simulink model "gm_sampleModel1655_sub"  (R2023a)
settings: Solver=VariableStepAuto  StartTime=0.0  StopTime=10.0  RelTol=1e-3
libraries: simulink x1
settings Model: Creator=user1  LastModifiedBy=user1
settings OptimizationCC: BlockReduction=off  ConditionallyExecuteInputs=off
settings DebuggingCC: InheritedTsInSrcMsg=none

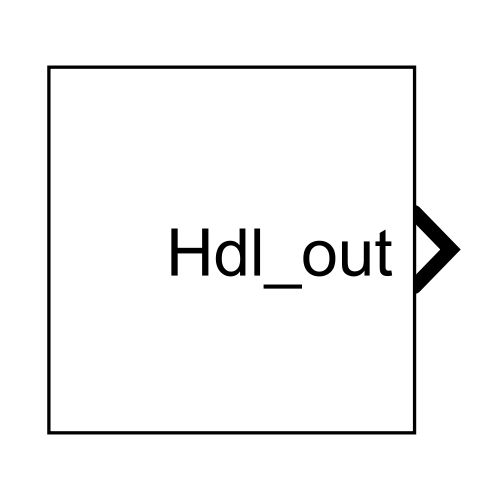
[thumbnail: Simulink's stored preview of the top-level diagram]
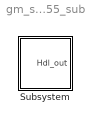
== system gm_sampleModel1655_sub ==
  Subsystem : Subsystem

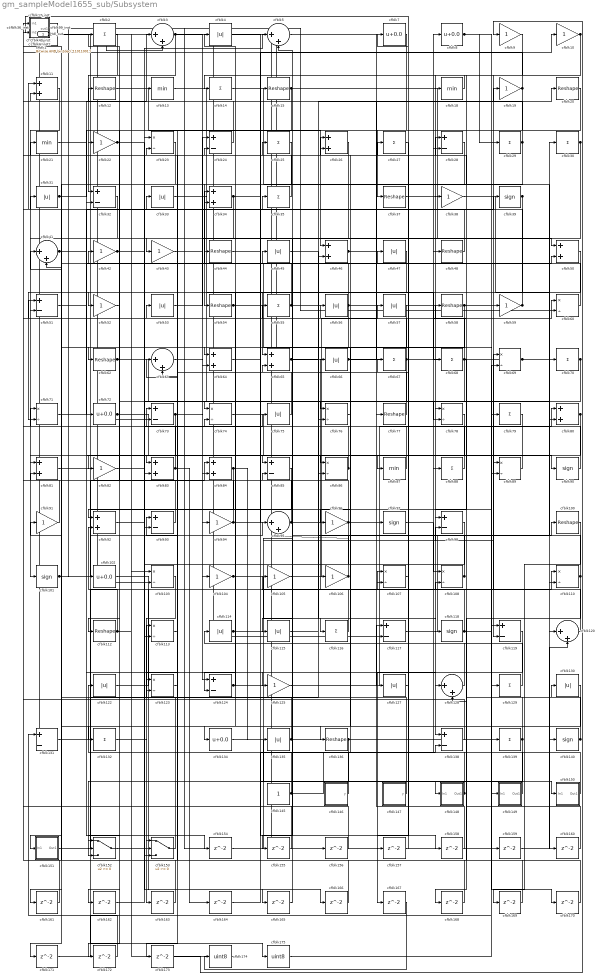
== system gm_sampleModel1655_sub/Subsystem ==
  cfblk1 : simulink/Logic and Bit Operations/Bitwise Operator  logicop=AND  UseBitMask=on  BitMask=bin2dec('11011001')  BitMaskRealWorld=Stored Integer
      settings: LibrarySourceBlock=|
      | hdlsllib/Logic and Bit
      | Operations/Bitwise
      | Operator
  cfblk{9..10,19,22,38,42..43,52,59,82,91,94,96,104..106,125} (17 alike) : Gain  OutDataTypeStr=uint8
  cfblk{12,15,20,37,44,48,54,58,62,77,100,112,136} (13 alike) : Reshape
  cfblk{39,90,97,101,118,140} (6 alike) : Signum
  cfblk{7..8,72,102,134} (5 alike) : Bias  Bias=0.0  SaturateOnIntegerOverflow=off
  cfblk{23,60,69,71,74,76,78,86,89,103,107..108,110,113,123} (15 alike) : Product  Inputs=*/  OutDataTypeStr=uint8  RndMeth=Zero  SaturateOnIntegerOverflow=on
  cfblk109_inst : Subsystem
  cfblk{11,26,34,46,50,64..65,80..81,83..84,92} (12 alike) : Sum  OutDataTypeStr=uint8
  cfblk{4,31,33,45,47,53,56..57,66,75,114..115,122,127,130,135} (16 alike) : Abs  OutDataTypeStr=uint8  SaturateOnIntegerOverflow=off
  cfblk{2,14,25,27,29..30,35,55,67..68,70,79,88,116,129,132,139} (17 alike) : Sum  Inputs=+  OutDataTypeStr=uint8
  cfblk{24,28,32,51,73,85,93,98,117,119,124,131,138} (13 alike) : Sum  Inputs=+-  OutDataTypeStr=uint8
  cfblk{3,5,41,63,95,120,128} (7 alike) : Sum  Inputs=|++  OutDataTypeStr=uint8
  cfblk121_inst : Subsystem
  cfblk{13,18,21,87} (4 alike) : MinMax  OutDataTypeStr=uint8
  cfblk133_inst : Subsystem
  cfblk137_inst : Subsystem
  cfblk145 : Constant  OutDataTypeStr=uint8  SampleTime=-1
  cfblk146 : Subsystem  mask(Counter Limited){uplimit=double(7), tsamp=double(-1)}
      mask prompts: uplimit "Simulink:masks:UpperLimit_MP"; tsamp "Simulink:masks:SampleTime_MP"
      mask help: Simulink:masks:CounterLimited_MD
      mask init:
      | nbits = double(8);
      | tsamp = double(-1);
      | uplimit = double(7);
  cfblk147 : Subsystem  mask(Counter Free-Running){NumBits=double(16), tsamp=double(-1)}
      mask prompts: NumBits "Simulink:masks:NumberOfBits_MP"; tsamp "Simulink:masks:SampleTime_MP"
      mask help: Simulink:masks:CounterFreeRunning_MD
  cfblk148 : Subsystem
  cfblk149 : Subsystem
  cfblk150 : Subsystem
  cfblk151 : Subsystem
  cfblk152 : Switch  OutDataTypeStr=uint8  SaturateOnIntegerOverflow=off  InputSameDT=off
  cfblk153 : Switch  OutDataTypeStr=uint8  SaturateOnIntegerOverflow=off  InputSameDT=off
  cfblk{154..173} (20 alike) : Delay  SampleTime=1
  cfblk16_inst : Subsystem
  cfblk174 : DataTypeConversion  OutDataTypeStr=uint8  SaturateOnIntegerOverflow=off  RndMeth=Floor
  cfblk175 : DataTypeConversion  OutDataTypeStr=uint8  SaturateOnIntegerOverflow=off  RndMeth=Floor
  cfblk17_inst : Subsystem
  cfblk36_inst : Subsystem
  cfblk40_inst : Subsystem
  cfblk6_inst : Subsystem
  cfblk99_inst : Subsystem
  Hdl_out : Outport  OutDataTypeStr=uint8  SampleTime=1
  wires:
  cfblk1/1 -> cfblk175/1
  cfblk10/1 -> cfblk138/1, cfblk119/2
  cfblk100/1 -> cfblk169/1
  cfblk101/1 -> cfblk95/1, cfblk84/1
  cfblk102/1 -> cfblk165/1
  cfblk103/1 -> cfblk163/1
  cfblk104/1 -> cfblk5/2, cfblk116/1
  cfblk105/1 -> cfblk57/1
  cfblk106/1 -> cfblk95/2, cfblk85/2
  cfblk107/1 -> cfblk99_inst/2(in2)
  cfblk108/1 -> cfblk121_inst/2(in2), cfblk42/1
  cfblk109_inst/1(out1) -> cfblk131/2
  cfblk11/1 -> cfblk101/1
  cfblk110/1 -> cfblk71/1, cfblk168/1
  cfblk112/1 -> cfblk92/2, cfblk103/1
  cfblk113/1 -> cfblk23/2
  cfblk114/1 -> cfblk98/2, cfblk69/1
  cfblk115/1 -> cfblk100/1
  cfblk116/1 -> cfblk105/1
  cfblk117/1 -> cfblk30/1
  cfblk118/1 -> cfblk66/1, cfblk58/1, cfblk170/1
  cfblk119/1 -> cfblk167/1
  cfblk12/1 -> cfblk46/1
  cfblk120/1 -> cfblk35/1
  cfblk121_inst/1(out1) -> cfblk159/1
  cfblk122/1 -> cfblk48/1
  cfblk123/1 -> cfblk33/1
  cfblk124/1 -> cfblk4/1, cfblk88/1
  cfblk125/1 -> cfblk80/1
  cfblk127/1 -> cfblk47/1
  cfblk128/1 -> cfblk7/1
  cfblk129/1 -> cfblk114/1
  cfblk13/1 -> cfblk78/1
  cfblk130/1 -> cfblk151/1(In1)
  cfblk131/1 -> cfblk107/1
  cfblk132/1 -> cfblk153/1
  cfblk133_inst/1(out1) -> cfblk6_inst/2(in2), cfblk117/2
  cfblk134/1 -> cfblk148/1(In1)
  cfblk135/1 -> cfblk53/1, cfblk21/1
  cfblk136/1 -> cfblk152/3, cfblk60/1, cfblk110/1
  cfblk137_inst/1(out1) -> cfblk102/1
  cfblk138/1 -> cfblk17_inst/1(in1)
  cfblk139/1 -> cfblk26/1, cfblk162/1
  cfblk14/1 -> cfblk80/2
  cfblk140/1 -> cfblk24/2, cfblk130/1
  cfblk145/1 -> cfblk8/1, cfblk63/2
  cfblk146/1(y) -> cfblk45/1
  cfblk147/1(y) -> cfblk113/1
  cfblk148/1(Out1) -> cfblk56/1, cfblk67/1
  cfblk149/1(Out1) -> cfblk122/1
  cfblk15/1 -> cfblk119/1, cfblk52/1
  cfblk150/1(Out1) -> cfblk93/1
  cfblk151/1(Out1) -> cfblk46/2
  cfblk152/1 -> cfblk5/1
  cfblk153/1 -> cfblk91/1
  cfblk154/1 -> cfblk89/1
  cfblk155/1 -> cfblk16_inst/2(in2)
  cfblk156/1 -> cfblk81/2
  cfblk157/1 -> cfblk107/2
  cfblk158/1 -> cfblk117/1
  cfblk159/1 -> cfblk120/2
  cfblk16_inst/1(out1) -> cfblk59/1
  cfblk160/1 -> cfblk28/1
  cfblk161/1 -> cfblk17_inst/2(in2)
  cfblk162/1 -> cfblk108/2
  cfblk163/1 -> cfblk133_inst/2(in2)
  cfblk164/1 -> cfblk138/2
  cfblk165/1 -> cfblk65/2
  cfblk166/1 -> cfblk73/1
  cfblk167/1 -> cfblk174/1
  cfblk168/1 -> cfblk99_inst/1(in1)
  cfblk169/1 -> cfblk11/2
  cfblk17_inst/1(out1) -> cfblk97/1
  cfblk170/1 -> cfblk128/2
  cfblk171/1 -> cfblk69/2
  cfblk172/1 -> cfblk131/1
  cfblk173/1 -> cfblk9/1
  cfblk174/1 -> cfblk1/1
  cfblk175/1 -> cfblk89/2
  cfblk18/1 -> cfblk14/1
  cfblk19/1 -> cfblk137_inst/2(in2), cfblk123/2, cfblk18/1
  cfblk2/1 -> cfblk32/1
  cfblk20/1 -> cfblk32/2
  cfblk21/1 -> cfblk72/1
  cfblk22/1 -> cfblk93/2, cfblk90/1
  cfblk23/1 -> cfblk62/1
  cfblk24/1 -> cfblk3/1
  cfblk25/1 -> cfblk54/1
  cfblk26/1 -> cfblk51/2
  cfblk27/1 -> cfblk157/1
  cfblk28/1 -> cfblk41/2
  cfblk29/1 -> cfblk84/2, cfblk109_inst/1(in1)
  cfblk3/1 -> cfblk50/1, cfblk22/1
  cfblk30/1 -> cfblk155/1, cfblk87/1
  cfblk31/1 -> cfblk83/1, cfblk13/1
  cfblk32/1 -> cfblk161/1
  cfblk33/1 -> cfblk68/1
  cfblk34/1 -> cfblk43/1, cfblk10/1
  cfblk35/1 -> cfblk16_inst/1(in1)
  cfblk36_inst/1(out1) -> cfblk103/2, cfblk139/1
  cfblk37/1 -> cfblk140/1
  cfblk38/1 -> cfblk70/1
  cfblk39/1 -> cfblk124/2, cfblk71/2
  cfblk4/1 -> cfblk150/1(In1)
  cfblk40_inst/1(out1) -> cfblk121_inst/1(in1), cfblk60/2
  cfblk41/1 -> cfblk50/2, cfblk125/1
  cfblk42/1 -> cfblk74/1, cfblk166/1
  cfblk43/1 -> cfblk24/1
  cfblk44/1 -> cfblk86/1
  cfblk45/1 -> cfblk106/1
  cfblk46/1 -> cfblk127/1, cfblk78/2
  cfblk47/1 -> cfblk65/1
  cfblk48/1 -> cfblk40_inst/1(in1)
  cfblk5/1 -> cfblk77/1
  cfblk50/1 -> cfblk64/1
  cfblk51/1 -> cfblk154/1
  cfblk52/1 -> cfblk112/1
  cfblk53/1 -> cfblk39/1
  cfblk54/1 -> cfblk28/2, cfblk79/1
  cfblk55/1 -> cfblk36_inst/2(in2), cfblk20/1
  cfblk56/1 -> cfblk23/1, cfblk171/1
  cfblk57/1 -> cfblk64/2
  cfblk58/1 -> cfblk76/1, cfblk132/1
  cfblk59/1 -> cfblk31/1, cfblk11/1
  cfblk6_inst/1(out1) -> cfblk156/1
  cfblk60/1 -> cfblk34/1
  cfblk62/1 -> cfblk83/2, cfblk160/1, cfblk104/1
  cfblk63/1 -> cfblk128/1
  cfblk64/1 -> cfblk158/1
  cfblk65/1 -> cfblk118/1, cfblk25/1
  cfblk66/1 -> cfblk26/2, cfblk19/1
  cfblk67/1 -> cfblk41/1, cfblk96/1
  cfblk68/1 -> cfblk98/1, cfblk36_inst/1(in1), cfblk76/2
  cfblk69/1 -> cfblk120/1, Hdl_out/1
  cfblk7/1 -> cfblk37/1
  cfblk70/1 -> cfblk152/2, cfblk173/1
  cfblk71/1 -> cfblk34/2
  cfblk72/1 -> cfblk85/1, cfblk94/1
  cfblk73/1 -> cfblk124/1, cfblk172/1
  cfblk74/1 -> cfblk86/2
  cfblk75/1 -> cfblk51/1
  cfblk76/1 -> cfblk136/1
  cfblk77/1 -> cfblk55/1
  cfblk78/1 -> cfblk134/1
  cfblk79/1 -> cfblk123/1
  cfblk8/1 -> cfblk149/1(In1), cfblk29/1
  cfblk80/1 -> cfblk153/2, cfblk110/2
  cfblk81/1 -> cfblk129/1
  cfblk82/1 -> cfblk113/2
  cfblk83/1 -> cfblk137_inst/1(in1), cfblk164/1
  cfblk84/1 -> cfblk152/1, cfblk135/1
  cfblk85/1 -> cfblk92/1
  cfblk86/1 -> cfblk82/1, cfblk2/1
  cfblk87/1 -> cfblk109_inst/2(in2)
  cfblk88/1 -> cfblk63/1
  cfblk89/1 -> cfblk81/1
  cfblk9/1 -> cfblk38/1
  cfblk90/1 -> cfblk27/1
  cfblk91/1 -> cfblk40_inst/2(in2)
  cfblk92/1 -> cfblk75/1
  cfblk93/1 -> cfblk6_inst/1(in1)
  cfblk94/1 -> cfblk15/1, cfblk133_inst/1(in1)
  cfblk95/1 -> cfblk12/1, cfblk74/2
  cfblk96/1 -> cfblk44/1, cfblk153/3
  cfblk97/1 -> cfblk108/1
  cfblk98/1 -> cfblk115/1
  cfblk99_inst/1(out1) -> cfblk73/2, cfblk3/2

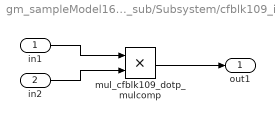
== system gm_sampleModel1655_sub/Subsystem/cfblk109_inst ==
  in1 : Inport  OutDataTypeStr=uint8  SampleTime=1
  in2 : Inport  Port=2  OutDataTypeStr=uint8  SampleTime=1
  mul_cfblk109_dotp_mulcomp : Product  Inputs=**  OutDataTypeStr=uint8  SampleTime=1
  out1 : Outport  OutDataTypeStr=uint8  SampleTime=1
  wires:
  in1/1 -> mul_cfblk109_dotp_mulcomp/1
  in2/1 -> mul_cfblk109_dotp_mulcomp/2
  mul_cfblk109_dotp_mulcomp/1 -> out1/1

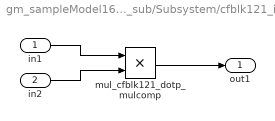
== system gm_sampleModel1655_sub/Subsystem/cfblk121_inst ==
  in1 : Inport  OutDataTypeStr=uint8  SampleTime=1
  in2 : Inport  Port=2  OutDataTypeStr=uint8  SampleTime=1
  mul_cfblk121_dotp_mulcomp : Product  Inputs=**  OutDataTypeStr=uint8  SampleTime=1
  out1 : Outport  OutDataTypeStr=uint8  SampleTime=1
  wires:
  in1/1 -> mul_cfblk121_dotp_mulcomp/1
  in2/1 -> mul_cfblk121_dotp_mulcomp/2
  mul_cfblk121_dotp_mulcomp/1 -> out1/1

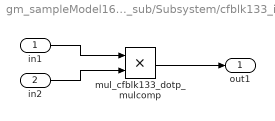
== system gm_sampleModel1655_sub/Subsystem/cfblk133_inst ==
  in1 : Inport  OutDataTypeStr=uint8  SampleTime=1
  in2 : Inport  Port=2  OutDataTypeStr=uint8  SampleTime=1
  mul_cfblk133_dotp_mulcomp : Product  Inputs=**  OutDataTypeStr=uint8  SampleTime=1
  out1 : Outport  OutDataTypeStr=uint8  SampleTime=1
  wires:
  in1/1 -> mul_cfblk133_dotp_mulcomp/1
  in2/1 -> mul_cfblk133_dotp_mulcomp/2
  mul_cfblk133_dotp_mulcomp/1 -> out1/1

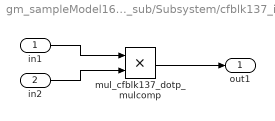
== system gm_sampleModel1655_sub/Subsystem/cfblk137_inst ==
  in1 : Inport  OutDataTypeStr=uint8  SampleTime=1
  in2 : Inport  Port=2  OutDataTypeStr=uint8  SampleTime=1
  mul_cfblk137_dotp_mulcomp : Product  Inputs=**  OutDataTypeStr=uint8  SampleTime=1
  out1 : Outport  OutDataTypeStr=uint8  SampleTime=1
  wires:
  in1/1 -> mul_cfblk137_dotp_mulcomp/1
  in2/1 -> mul_cfblk137_dotp_mulcomp/2
  mul_cfblk137_dotp_mulcomp/1 -> out1/1

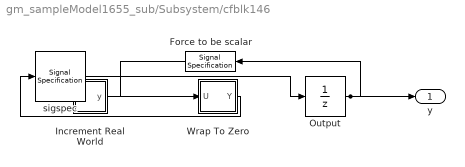
== system gm_sampleModel1655_sub/Subsystem/cfblk146 ==
  Force to be scalar : SignalSpecification  DisableCoverage=on  Dimensions=1
  Increment Real World : Subsystem  mask(Real World Value Increment){}
      mask help: Simulink:masks:RealWorldValueIncrement_MD
      mask Display: disp('V++')
  Output : UnitDelay  InitialCondition=0.0  SampleTime=tsamp  HasFrameUpgradeWarning=on
  Wrap To Zero : Subsystem  mask(Wrap To Zero){Threshold=double(7)}
      mask prompts: Threshold "Simulink:masks:Threshold_MP"
      mask help: Simulink:masks:WrapToZero_MD
  sigspec : SignalSpecification  OutDataTypeStr=uint8  Dimensions=1
  y : Outport  SampleTime=1
  wires:
  Force to be scalar/1 -> Increment Real World/1(u)
  Increment Real World/1(y) -> Wrap To Zero/1(U)
  Output/1 -> Force to be scalar/1, y/1
  Wrap To Zero/1(Y) -> sigspec/1
  sigspec/1 -> Output/1

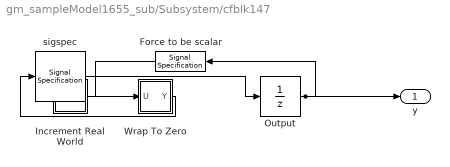
== system gm_sampleModel1655_sub/Subsystem/cfblk147 ==
  Force to be scalar : SignalSpecification  DisableCoverage=on  Dimensions=1
  Increment Real World : Subsystem  mask(Real World Value Increment){}
      mask help: Simulink:masks:RealWorldValueIncrement_MD
      mask Display: disp('V++')
  Output : UnitDelay  InitialCondition=0.0  SampleTime=tsamp  HasFrameUpgradeWarning=on
  Wrap To Zero : Subsystem  mask(Wrap To Zero){Threshold=double(65535)}
      mask prompts: Threshold "Simulink:masks:Threshold_MP"
      mask help: Simulink:masks:WrapToZero_MD
  sigspec : SignalSpecification  OutDataTypeStr=uint16  Dimensions=1
  y : Outport  SampleTime=1
  wires:
  Force to be scalar/1 -> Increment Real World/1(u)
  Increment Real World/1(y) -> Wrap To Zero/1(U)
  Output/1 -> Force to be scalar/1, y/1
  Wrap To Zero/1(Y) -> sigspec/1
  sigspec/1 -> Output/1

== system gm_sampleModel1655_sub/Subsystem/cfblk148 ==
  In1 : Inport  OutDataTypeStr=uint8  PortDimensions=1  SampleTime=1
  Out1 : Outport  SampleTime=1
  wires:
  In1/1 -> Out1/1

== system gm_sampleModel1655_sub/Subsystem/cfblk149 ==
  In1 : Inport  OutDataTypeStr=uint8  PortDimensions=1  SampleTime=1
  Out1 : Outport  SampleTime=1
  wires:
  In1/1 -> Out1/1

== system gm_sampleModel1655_sub/Subsystem/cfblk150 ==
  In1 : Inport  OutDataTypeStr=uint8  PortDimensions=1  SampleTime=1
  Out1 : Outport  SampleTime=1
  wires:
  In1/1 -> Out1/1

== system gm_sampleModel1655_sub/Subsystem/cfblk151 ==
  In1 : Inport  OutDataTypeStr=uint8  PortDimensions=1  SampleTime=1
  Out1 : Outport  SampleTime=1
  wires:
  In1/1 -> Out1/1

== system gm_sampleModel1655_sub/Subsystem/cfblk16_inst ==
  in1 : Inport  OutDataTypeStr=uint8  SampleTime=1
  in2 : Inport  Port=2  OutDataTypeStr=uint8  SampleTime=1
  mul_cfblk16_dotp_mulcomp : Product  Inputs=**  OutDataTypeStr=uint8  SampleTime=1
  out1 : Outport  OutDataTypeStr=uint8  SampleTime=1
  wires:
  in1/1 -> mul_cfblk16_dotp_mulcomp/1
  in2/1 -> mul_cfblk16_dotp_mulcomp/2
  mul_cfblk16_dotp_mulcomp/1 -> out1/1

== system gm_sampleModel1655_sub/Subsystem/cfblk17_inst ==
  in1 : Inport  OutDataTypeStr=uint8  SampleTime=1
  in2 : Inport  Port=2  OutDataTypeStr=uint8  SampleTime=1
  mul_cfblk17_dotp_mulcomp : Product  Inputs=**  OutDataTypeStr=uint8  SampleTime=1
  out1 : Outport  OutDataTypeStr=uint8  SampleTime=1
  wires:
  in1/1 -> mul_cfblk17_dotp_mulcomp/1
  in2/1 -> mul_cfblk17_dotp_mulcomp/2
  mul_cfblk17_dotp_mulcomp/1 -> out1/1

== system gm_sampleModel1655_sub/Subsystem/cfblk36_inst ==
  in1 : Inport  OutDataTypeStr=uint8  SampleTime=1
  in2 : Inport  Port=2  OutDataTypeStr=uint8  SampleTime=1
  mul_cfblk36_dotp_mulcomp : Product  Inputs=**  OutDataTypeStr=uint8  SampleTime=1
  out1 : Outport  OutDataTypeStr=uint8  SampleTime=1
  wires:
  in1/1 -> mul_cfblk36_dotp_mulcomp/1
  in2/1 -> mul_cfblk36_dotp_mulcomp/2
  mul_cfblk36_dotp_mulcomp/1 -> out1/1

== system gm_sampleModel1655_sub/Subsystem/cfblk40_inst ==
  in1 : Inport  OutDataTypeStr=uint8  SampleTime=1
  in2 : Inport  Port=2  OutDataTypeStr=uint8  SampleTime=1
  mul_cfblk40_dotp_mulcomp : Product  Inputs=**  OutDataTypeStr=uint8  SampleTime=1
  out1 : Outport  OutDataTypeStr=uint8  SampleTime=1
  wires:
  in1/1 -> mul_cfblk40_dotp_mulcomp/1
  in2/1 -> mul_cfblk40_dotp_mulcomp/2
  mul_cfblk40_dotp_mulcomp/1 -> out1/1

== system gm_sampleModel1655_sub/Subsystem/cfblk6_inst ==
  in1 : Inport  OutDataTypeStr=uint8  SampleTime=1
  in2 : Inport  Port=2  OutDataTypeStr=uint8  SampleTime=1
  mul_cfblk6_dotp_mulcomp : Product  Inputs=**  OutDataTypeStr=uint8  SampleTime=1
  out1 : Outport  OutDataTypeStr=uint8  SampleTime=1
  wires:
  in1/1 -> mul_cfblk6_dotp_mulcomp/1
  in2/1 -> mul_cfblk6_dotp_mulcomp/2
  mul_cfblk6_dotp_mulcomp/1 -> out1/1

== system gm_sampleModel1655_sub/Subsystem/cfblk99_inst ==
  in1 : Inport  OutDataTypeStr=uint8  SampleTime=1
  in2 : Inport  Port=2  OutDataTypeStr=uint8  SampleTime=1
  mul_cfblk99_dotp_mulcomp : Product  Inputs=**  OutDataTypeStr=uint8  SampleTime=1
  out1 : Outport  OutDataTypeStr=uint8  SampleTime=1
  wires:
  in1/1 -> mul_cfblk99_dotp_mulcomp/1
  in2/1 -> mul_cfblk99_dotp_mulcomp/2
  mul_cfblk99_dotp_mulcomp/1 -> out1/1

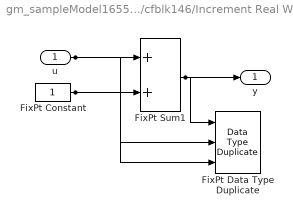
== system gm_sampleModel1655_sub/Subsystem/cfblk146/Increment Real World ==
  u : Inport  OutDataTypeStr=uint8  SampleTime=1
  FixPt Constant : Constant  DisableCoverage=on  OutDataTypeStr=Inherit: Inherit via back propagation  SampleTime=-1
  FixPt Data Type Duplicate : DataTypeDuplicate  DisableCoverage=on  NumInputPorts=3
  FixPt Sum1 : Sum  InputSameDT=on  OutDataTypeStr=Inherit: Inherit via back propagation  LockScale=on
  y : Outport  SampleTime=1
  wires:
  u/1 -> FixPt Sum1/1, FixPt Data Type Duplicate/2
  FixPt Constant/1 -> FixPt Sum1/2, FixPt Data Type Duplicate/3
  FixPt Sum1/1 -> FixPt Data Type Duplicate/1, y/1

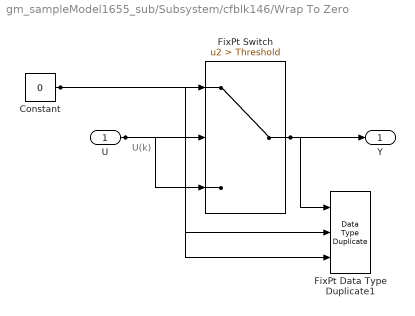
== system gm_sampleModel1655_sub/Subsystem/cfblk146/Wrap To Zero ==
  note: U(k)
  U : Inport  OutDataTypeStr=uint8  SampleTime=1
  Constant : Constant  DisableCoverage=on  Value=0  OutDataTypeStr=Inherit: Inherit via back propagation  SampleTime=-1
  FixPt Data Type Duplicate1 : DataTypeDuplicate  DisableCoverage=on  NumInputPorts=3
  FixPt Switch : Switch  Criteria=u2 > Threshold  Threshold=Threshold  OutDataTypeStr=Inherit: Inherit via back propagation  ZeroCross=off  SaturateOnIntegerOverflow=off  InputSameDT=off
  Y : Outport  SampleTime=1
  wires:
  U/1 -> FixPt Switch/3, FixPt Switch/2, FixPt Data Type Duplicate1/2
  Constant/1 -> FixPt Switch/1, FixPt Data Type Duplicate1/3
  FixPt Switch/1 -> FixPt Data Type Duplicate1/1, Y/1

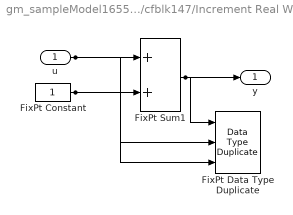
== system gm_sampleModel1655_sub/Subsystem/cfblk147/Increment Real World ==
  u : Inport  OutDataTypeStr=uint16  SampleTime=1
  FixPt Constant : Constant  DisableCoverage=on  OutDataTypeStr=Inherit: Inherit via back propagation  SampleTime=-1
  FixPt Data Type Duplicate : DataTypeDuplicate  DisableCoverage=on  NumInputPorts=3
  FixPt Sum1 : Sum  InputSameDT=on  OutDataTypeStr=Inherit: Inherit via back propagation  LockScale=on
  y : Outport  SampleTime=1
  wires:
  u/1 -> FixPt Sum1/1, FixPt Data Type Duplicate/2
  FixPt Constant/1 -> FixPt Sum1/2, FixPt Data Type Duplicate/3
  FixPt Sum1/1 -> FixPt Data Type Duplicate/1, y/1

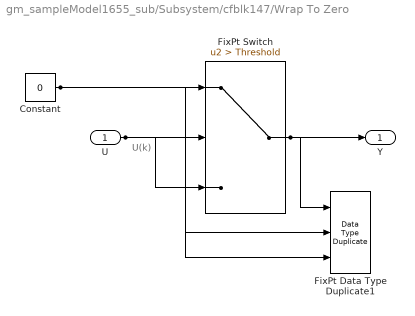
== system gm_sampleModel1655_sub/Subsystem/cfblk147/Wrap To Zero ==
  note: U(k)
  U : Inport  OutDataTypeStr=uint16  SampleTime=1
  Constant : Constant  DisableCoverage=on  Value=0  OutDataTypeStr=Inherit: Inherit via back propagation  SampleTime=-1
  FixPt Data Type Duplicate1 : DataTypeDuplicate  DisableCoverage=on  NumInputPorts=3
  FixPt Switch : Switch  Criteria=u2 > Threshold  Threshold=Threshold  OutDataTypeStr=Inherit: Inherit via back propagation  ZeroCross=off  SaturateOnIntegerOverflow=off  InputSameDT=off
  Y : Outport  SampleTime=1
  wires:
  U/1 -> FixPt Switch/3, FixPt Switch/2, FixPt Data Type Duplicate1/2
  Constant/1 -> FixPt Switch/1, FixPt Data Type Duplicate1/3
  FixPt Switch/1 -> FixPt Data Type Duplicate1/1, Y/1
